simulink model "platformController"  (R2025b)
settings: Solver=FixedStepDiscrete  StartTime=0.0  StopTime=10  FixedStep=1/1000  RelTol=1e-3
InitFcn:
  | plant_parameters;
  | fluid_constants;
undefined symbols (not defined in the file or in its folder): DiscIntNeverNeededParam, mass, mission_mode, platform_targets
libraries: simulink x12, slpidlib x3, eeGeneralControl x1
settings Model: Creator=karadeli  LastModifiedBy=karadeli
settings OptimizationCC: DefaultParameterBehavior=Inlined  UseDivisionForNetSlopeComputation=on  GainParamInheritBuiltInType=on  UseFloatMulNetSlope=on  InlineInvariantSignals=on  PassReuseOutputArgsAs=Individual arguments  ZeroExternalMemoryAtStartup=off  ZeroInternalMemoryAtStartup=off  NoFixptDivByZeroProtection=on  EfficientFloat2IntCast=on  LifeSpan=1  OptimizeBlockOrder=speed  DifferentSizesBufferReuse=on  EfficientTunableParamExpr=on
settings DebuggingCC: ParameterTunabilityLossMsg=error
settings HardwareCC: ProdBitPerPointer=32.0  ProdBitPerSizeT=32.0  ProdBitPerPtrDiffT=32.0  ProdLargestAtomicInteger=Long  ProdLargestAtomicFloat=Double  ProdWordSize=32.0  ProdLongLongMode=on  ProdHWDeviceType=ARM Compatible->ARM Cortex-M
settings SFSimCC: MATLABDynamicMemAlloc=off
settings RTWCC: SystemTargetFile=ert.tlc  GenCodeOnly=on  TemplateMakefile=ert_default_tmf  TargetLang=C++  Description=Embedded Coder
settings CodeAppCC: ForceParamTrailComments=on  IgnoreCustomStorageClasses=off  OperatorAnnotations=on  SimulinkDataObjDesc=on  SFDataObjDesc=on  CustomSymbolStrGlobalVar=rt$N$M  CustomSymbolStrType=$N$M  CustomSymbolStrFcn=$N$M$F  CustomSymbolStrMacro=$N$M  InsertBlockDesc=on
settings ERTTargetCC: RootIOFormat=Structure reference  ERTCustomFileTemplate=example_file_process.tlc  ERTFilePackagingFormat=CompactWithDataFile  TargetLangStandard=C++11 (ISO)  GenerateSampleERTMain=on  IncludeMdlTerminateFcn=off  CombineSignalStateStructs=on  SupportAbsoluteTime=off  CodeInterfacePackaging=C++ class  SubcomponentCodeInterfacePackaging=C++ class  SupportNonFinite=off  SupportComplex=off  SupportNonInlinedSFcns=on

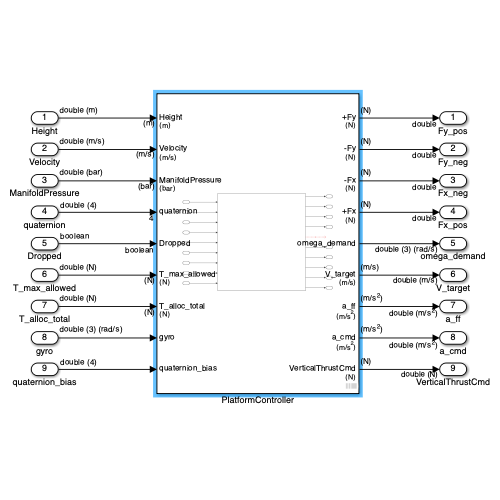
[thumbnail: Simulink's stored preview of the top-level diagram]
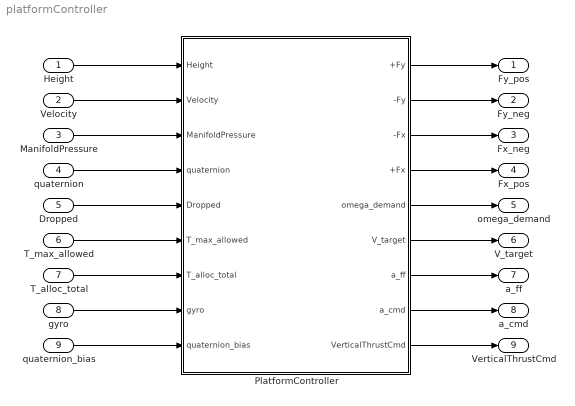
== system platformController ==
  Height : Inport  Unit=m
  Velocity : Inport  Port=2  Unit=m/s
  ManifoldPressure : Inport  Port=3  Unit=bar
  quaternion : Inport  Port=4  PortDimensions=4
  Dropped : Inport  Port=5  OutDataTypeStr=boolean
  T_max_allowed : Inport  Port=6  Unit=N
  T_alloc_total : Inport  Port=7  Unit=N
  gyro : Inport  Port=8
  quaternion_bias : Inport  Port=9  PortDimensions=4
  PlatformController : Subsystem
  Fy_pos : Outport
  Fy_neg : Outport  Port=2
  Fx_neg : Outport  Port=3
  Fx_pos : Outport  Port=4
  omega_demand : Outport  Port=5
  V_target : Outport  Port=6  Unit=m/s
  a_ff : Outport  Port=7  Unit=m/s^2
  a_cmd : Outport  Port=8  Unit=m/s^2
  VerticalThrustCmd : Outport  Port=9  Unit=N
  wires:
  T_max_allowed/1 -> PlatformController/6(T_max_allowed)
  T_alloc_total/1 -> PlatformController/7(T_alloc_total)
  Height/1 -> PlatformController/1(Height)
  Velocity/1 -> PlatformController/2(Velocity)
  quaternion/1 -> PlatformController/4(quaternion)
  ManifoldPressure/1 -> PlatformController/3(ManifoldPressure)
  Dropped/1 -> PlatformController/5(Dropped)
  gyro/1 -> PlatformController/8(gyro)
  PlatformController/5(omega_demand) -> omega_demand/1
  PlatformController/4(+Fx) -> Fx_pos/1
  PlatformController/3(-Fx) -> Fx_neg/1
  PlatformController/2(-Fy) -> Fy_neg/1
  PlatformController/1(+Fy) -> Fy_pos/1
  quaternion_bias/1 -> PlatformController/9(quaternion_bias)
  PlatformController/6(V_target) -> V_target/1
  PlatformController/9(VerticalThrustCmd) -> VerticalThrustCmd/1
  PlatformController/8(a_cmd) -> a_cmd/1
  PlatformController/7(a_ff) -> a_ff/1

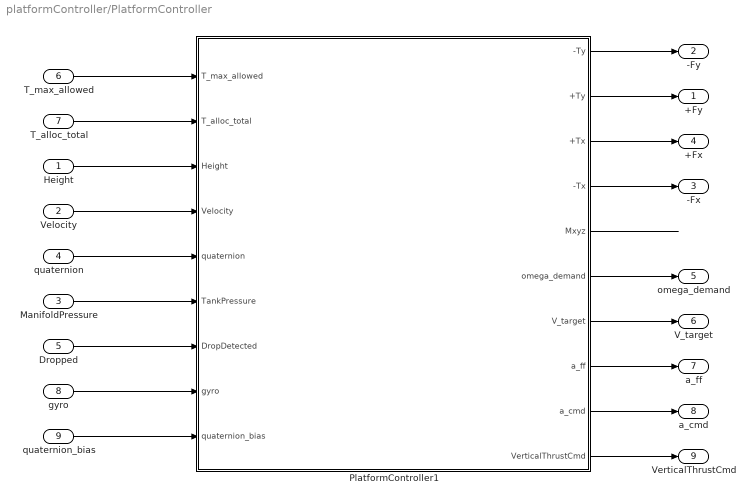
== system platformController/PlatformController ==
  Height : Inport  Unit=m
  Velocity : Inport  Port=2  Unit=m/s
  ManifoldPressure : Inport  Port=3  Unit=bar
  quaternion : Inport  Port=4  PortDimensions=4
  Dropped : Inport  Port=5  OutDataTypeStr=boolean
  T_max_allowed : Inport  Port=6  Unit=N
  T_alloc_total : Inport  Port=7  Unit=N
  gyro : Inport  Port=8
  quaternion_bias : Inport  Port=9
  PlatformController1 : Subsystem
  +Fy : Outport  Unit=N
  -Fy : Outport  Port=2  Unit=N
  -Fx : Outport  Port=3  Unit=N
  +Fx : Outport  Port=4  Unit=N
  omega_demand : Outport  Port=5
  V_target : Outport  Port=6  Unit=m/s
  a_ff : Outport  Port=7  Unit=m/s^2
  a_cmd : Outport  Port=8  Unit=m/s^2
  VerticalThrustCmd : Outport  Port=9  Unit=N
  wires:
  PlatformController1/1(-Ty) -> -Fy/1
  Height/1 -> PlatformController1/3(Height)
  gyro/1 -> PlatformController1/8(gyro)
  PlatformController1/6(omega_demand) -> omega_demand/1
  PlatformController1/5(Mxyz) -> ?
  Dropped/1 -> PlatformController1/7(DropDetected)
  T_alloc_total/1 -> PlatformController1/2(T_alloc_total)
  PlatformController1/2(+Ty) -> +Fy/1
  PlatformController1/4(-Tx) -> -Fx/1
  T_max_allowed/1 -> PlatformController1/1(T_max_allowed)
  quaternion/1 -> PlatformController1/5(quaternion)
  Velocity/1 -> PlatformController1/4(Velocity)
  ManifoldPressure/1 -> PlatformController1/6(TankPressure)
  PlatformController1/3(+Tx) -> +Fx/1
  quaternion_bias/1 -> PlatformController1/9(quaternion_bias)
  PlatformController1/7(V_target) -> V_target/1
  PlatformController1/8(a_ff) -> a_ff/1
  PlatformController1/9(a_cmd) -> a_cmd/1
  PlatformController1/10(VerticalThrustCmd) -> VerticalThrustCmd/1

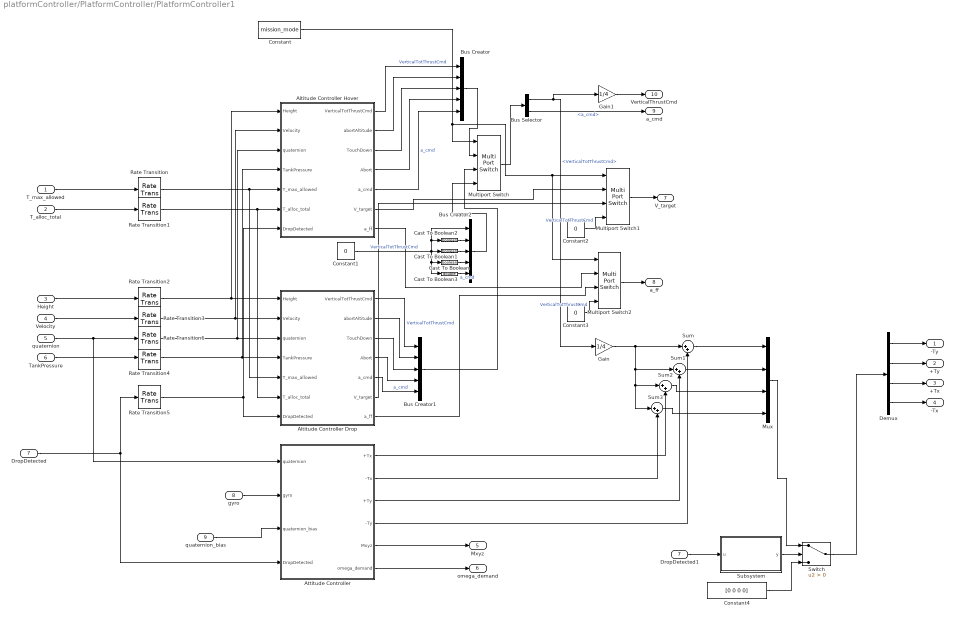
== system platformController/PlatformController/PlatformController1 ==
  T_max_allowed : Inport
  T_alloc_total : Inport  Port=2
  Height : Inport  Port=3
  Velocity : Inport  Port=4
  quaternion : Inport  Port=5
  TankPressure : Inport  Port=6
  DropDetected : Inport  Port=7
  gyro : Inport  Port=8  Unit=rad/s  PortDimensions=3
  quaternion_bias : Inport  Port=9
  Altitude Controller Drop : Subsystem
  Altitude Controller Hover : Subsystem
  Attitude Controller : Subsystem
  Bus Creator : BusCreator  Inputs=5
  Bus Creator1 : BusCreator  Inputs=5
  Bus Creator2 : BusCreator  Inputs=5
  Bus Selector : BusSelector  OutputSignals=VerticalTotThrustCmd,a_cmd
  Cast To Boolean : DataTypeConversion  OutDataTypeStr=boolean  SaturateOnIntegerOverflow=off  RndMeth=Floor
  Cast To Boolean1 : DataTypeConversion  OutDataTypeStr=boolean  SaturateOnIntegerOverflow=off  RndMeth=Floor
  Cast To Boolean2 : DataTypeConversion  OutDataTypeStr=boolean  SaturateOnIntegerOverflow=off  RndMeth=Floor
  Cast To Boolean3 : DataTypeConversion  OutDataTypeStr=double  SaturateOnIntegerOverflow=off  RndMeth=Floor
  Constant : Constant  Value=mission_mode  OutDataTypeStr=Enum: mission_modes
  Constant1 : Constant  Value=0
  Constant2 : Constant  Value=0
  Constant3 : Constant  Value=0
  Constant4 : Constant  Value=[0 0 0 0]
  Demux : Demux
  DropDetected1 : InportShadow  Port=7
  Gain : Gain  Gain=1/4
  Gain1 : Gain  Gain=1/4
  Multiport Switch : MultiPortSwitch  DataPortOrder=Specify indices  DataPortIndices={mission_modes.HOVER, mission_modes.DROP}  DataPortForDefault=Additional data port  SaturateOnIntegerOverflow=off  InputSameDT=off
  Multiport Switch1 : MultiPortSwitch  DataPortOrder=Specify indices  DataPortIndices={mission_modes.HOVER, mission_modes.DROP}  DataPortForDefault=Additional data port  SaturateOnIntegerOverflow=off  InputSameDT=off
  Multiport Switch2 : MultiPortSwitch  DataPortOrder=Specify indices  DataPortIndices={mission_modes.HOVER, mission_modes.DROP}  DataPortForDefault=Additional data port  SaturateOnIntegerOverflow=off  InputSameDT=off
  Mux : Mux
  Rate Transition{,1..6} (7 alike) : RateTransition  OutPortSampleTime=1/50
  Subsystem : Subsystem  mask{t_close=5}
  Sum{,1..3} (4 alike) : Sum  Inputs=|++
  Switch : Switch  Criteria=u2 > Threshold  SaturateOnIntegerOverflow=off  InputSameDT=off
  -Ty : Outport
  +Ty : Outport  Port=2
  +Tx : Outport  Port=3
  -Tx : Outport  Port=4
  Mxyz : Outport  Port=5
  omega_demand : Outport  Port=6
  V_target : Outport  Port=7
  a_ff : Outport  Port=8
  a_cmd : Outport  Port=9
  VerticalThrustCmd : Outport  Port=10
  wires:
  Cast To Boolean1/1 -> Bus Creator2/3
  T_alloc_total/1 -> Rate Transition1/1
  Sum2/1 -> Mux/3
  T_max_allowed/1 -> Rate Transition/1
  Altitude Controller Hover/2(abortAltitude) -> Bus Creator/2
  Multiport Switch/1 -> Bus Selector/1
  Cast To Boolean/1 -> Bus Creator2/4
  Altitude Controller Hover/3(TouchDown) -> Bus Creator/3
  Attitude Controller/2(-Tx) -> Sum3/2
  quaternion/1 -> Rate Transition6/1, Attitude Controller/1(quaternion)
  Height/1 -> Rate Transition2/1
  Velocity/1 -> Rate Transition3/1
  Cast To Boolean3/1 -> Bus Creator2/5  "a_cmd"
  gyro/1 -> Attitude Controller/2(gyro)
  Altitude Controller Hover/1(VerticalTotThrustCmd) -> Bus Creator/1  "VerticalTotThrustCmd"
  Gain/1 -> Sum/1, Sum1/1, Sum3/1, Sum2/1
  Bus Selector/1 -> Gain1/1, Gain/1  "<VerticalTotThrustCmd>"
  TankPressure/1 -> Rate Transition4/1
  Altitude Controller Drop/4(Abort) -> Bus Creator1/4
  Constant1/1 -> Cast To Boolean1/1, Cast To Boolean/1, Cast To Boolean3/1, Cast To Boolean2/1, Bus Creator2/1  "VerticalTotThrustCmd"
  Attitude Controller/1(+Tx) -> Sum2/2
  Attitude Controller/3(+Ty) -> Sum1/2
  Altitude Controller Drop/1(VerticalTotThrustCmd) -> Bus Creator1/1  "VerticalTotThrustCmd"
  Bus Creator/1 -> Multiport Switch/2
  Attitude Controller/4(-Ty) -> Sum/2
  Bus Creator1/1 -> Multiport Switch/3
  Altitude Controller Hover/4(Abort) -> Bus Creator/4
  DropDetected/1 -> Rate Transition5/1, Attitude Controller/4(DropDetected)
  Altitude Controller Drop/3(TouchDown) -> Bus Creator1/3
  Sum/1 -> Mux/1
  Altitude Controller Drop/2(abortAltitude) -> Bus Creator1/2
  Altitude Controller Hover/5(a_cmd) -> Bus Creator/5  "a_cmd"
  Cast To Boolean2/1 -> Bus Creator2/2
  Constant/1 -> Multiport Switch/1, Multiport Switch1/1, Multiport Switch2/1
  Bus Creator2/1 -> Multiport Switch/4
  Altitude Controller Drop/5(a_cmd) -> Bus Creator1/5  "a_cmd"
  Sum1/1 -> Mux/2
  Sum3/1 -> Mux/4
  Attitude Controller/5(Mxyz) -> Mxyz/1
  Rate Transition/1 -> Altitude Controller Drop/5(T_max_allowed), Altitude Controller Hover/5(T_max_allowed)
  Rate Transition1/1 -> Altitude Controller Drop/6(T_alloc_total), Altitude Controller Hover/6(T_alloc_total)
  Rate Transition2/1 -> Altitude Controller Hover/1(Height), Altitude Controller Drop/1(Height)
  Rate Transition3/1 -> Altitude Controller Hover/2(Velocity), Altitude Controller Drop/2(Velocity)
  Rate Transition4/1 -> Altitude Controller Hover/4(TankPressure), Altitude Controller Drop/4(TankPressure)
  Rate Transition5/1 -> Altitude Controller Hover/7(DropDetected), Altitude Controller Drop/7(DropDetected)
  Rate Transition6/1 -> Altitude Controller Drop/3(quaternion), Altitude Controller Hover/3(quaternion)
  Attitude Controller/6(omega_demand) -> omega_demand/1
  quaternion_bias/1 -> Attitude Controller/3(quaternion_bias)
  Altitude Controller Hover/6(V_target) -> Multiport Switch1/2
  Altitude Controller Drop/6(V_target) -> Multiport Switch1/3
  Constant2/1 -> Multiport Switch1/4  "VerticalTotThrustCmd"
  Multiport Switch1/1 -> V_target/1
  Constant3/1 -> Multiport Switch2/4  "VerticalTotThrustCmd"
  Multiport Switch2/1 -> a_ff/1
  Altitude Controller Hover/7(a_ff) -> Multiport Switch2/2
  Altitude Controller Drop/7(a_ff) -> Multiport Switch2/3
  Bus Selector/2 -> a_cmd/1  "<a_cmd>"
  Gain1/1 -> VerticalThrustCmd/1
  DropDetected1/1 -> Subsystem/1(u)
  Subsystem/1(y) -> Switch/2
  Constant4/1 -> Switch/3
  Demux/2 -> +Ty/1
  Demux/4 -> -Tx/1
  Demux/3 -> +Tx/1
  Demux/1 -> -Ty/1
  Mux/1 -> Switch/1
  Switch/1 -> Demux/1

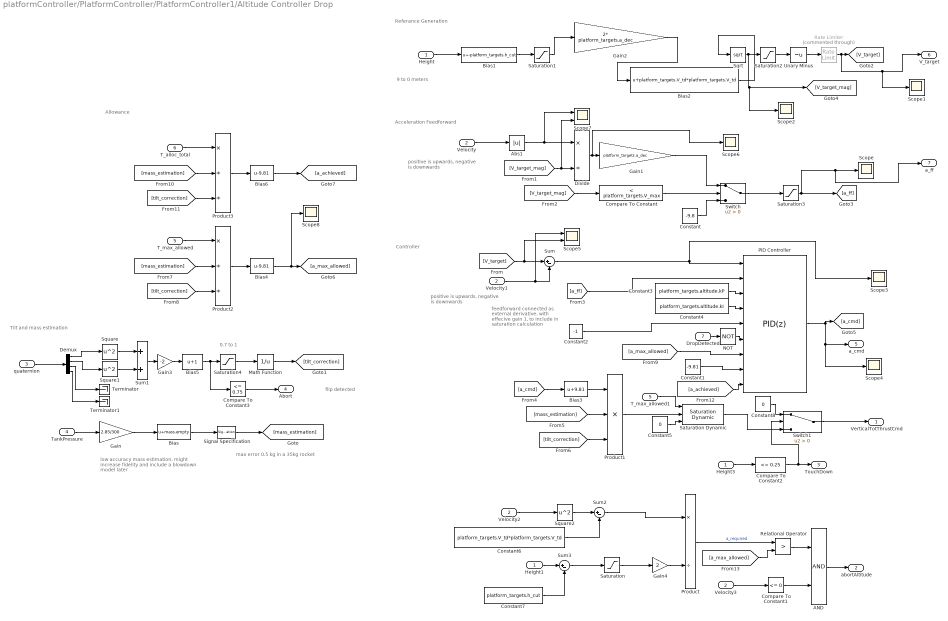
== system platformController/PlatformController/PlatformController1/Altitude Controller Drop ==
  note: flip detected
  note: max error 0.5 kg in a 35kg rocket
  note: 0.7 to 1
  note: Allowance
  note: Controller
  note: feedforward connected as external derivative, with effecive gain 1, to include in saturation calculation
  note: Tilt and mass estimation
  note: Acceleration Feedforward
  note: Referance Generation
  note: 9 to 0 meters
  note: low accuracy mass estimation, might increase fidelity and include a blowdown model later
  note: positive is upwards, negative is downwards
  note: positive is upwards, negative is downwards
  Height : Inport
  Velocity : Inport  Port=2
  quaternion : Inport  Port=3
  TankPressure : Inport  Port=4  Unit=bar
  T_max_allowed : Inport  Port=5  Unit=N
  T_alloc_total : Inport  Port=6
  DropDetected : Inport  Port=7
  AND : Logic  AllPortsSameDT=off  OutDataTypeStr=boolean
  Abs1 : Abs  SaturateOnIntegerOverflow=off
  Bias : Bias  Bias=mass.empty  SaturateOnIntegerOverflow=off
  Bias1 : Bias  Bias=-platform_targets.h_cut  SaturateOnIntegerOverflow=off
  Bias2 : Bias  Bias=platform_targets.V_td*platform_targets.V_td  SaturateOnIntegerOverflow=off
  Bias3 : Bias  Bias=9.81  SaturateOnIntegerOverflow=off
  Bias4 : Bias  Bias=-9.81  SaturateOnIntegerOverflow=off
  Bias5 : Bias  Bias=1  SaturateOnIntegerOverflow=off
  Bias6 : Bias  Bias=-9.81  SaturateOnIntegerOverflow=off
  Compare To Constant : simulink/Logic and Bit Operations/Compare To Constant  relop=<  const=platform_targets.V_max  OutDataTypeStr=boolean
  Compare To Constant1 : simulink/Logic and Bit Operations/Compare To Constant  relop=<=  const=0  OutDataTypeStr=boolean
  Compare To Constant2 : simulink/Logic and Bit Operations/Compare To Constant  relop=<=  const=0.25  OutDataTypeStr=boolean
  Compare To Constant3 : simulink/Logic and Bit Operations/Compare To Constant  relop=<=  const=0.75  OutDataTypeStr=boolean
  Constant : Constant  Value=-9.8
  Constant1 : Constant  Value=-9.81
  Constant2 : Constant  Value=-1
  Constant3 : Constant  Value=platform_targets.altitude.kP
  Constant4 : Constant  Value=platform_targets.altitude.kI
  Constant5 : Constant  Value=0
  Constant6 : Constant  Value=platform_targets.V_td*platform_targets.V_td
  Constant7 : Constant  Value=platform_targets.h_cut
  Constant8 : Constant  Value=0
  Demux : Demux
  Divide : Product  Inputs=*/
  Gain : Gain  Gain=2.85/300
  Gain1 : Gain  Gain=platform_targets.a_dec
  Gain2 : Gain  Gain=2* platform_targets.a_dec
  Gain3 : Gain  Gain=-2
  Gain4 : Gain  Gain=2
  Height1 : InportShadow
  Height3 : InportShadow
  Math Function : Math  Operator=reciprocal
  NOT : Logic  Operator=NOT  IconShape=distinctive  AllPortsSameDT=off  OutDataTypeStr=boolean
  PID Controller : slpidlib/PID Controller  Controller=PID  Form=Parallel  TimeDomain=Discrete-time  UseExternalTs=off  SampleTime=-1  IntegratorMethod=Forward Euler  FilterMethod=Forward Euler  ControllerParametersSource=external  P=1  I=1  UseKiTs=off  D=platform_targets.Ts  UseExternalDerivativeSource=on  N=100  UseFilter=off  TunerSelectOption=Frequency Response Based  InitialConditionSource=internal  InitialConditionForIntegrator=0  InitialConditionForFilter=0  DifferentiatorICPrevScaledInput=0  ExternalReset=level  TrackingMode=on  Kt=1  LimitOutput=on  SatLimitsSource=external  UpperSaturationLimit=inf  LowerSaturationLimit=-inf  LinearizeAsGain=on  AntiWindupMode=clamping  Kb=1  LimitIntegrator=on  UpperIntegratorSaturationLimit=3  LowerIntegratorSaturationLimit=-3  POutMin=[]  POutMax=[]  IOutMin=[]  IOutMax=[]  DOutMin=[]  DOutMax=[]  NOutMin=[]  NOutMax=[]  SumOutMin=[]  SumOutMax=[]  SaturationOutMin=[]  SaturationOutMax=[]  PParamMin=[]  PParamMax=[]  IParamMin=[]  IParamMax=[]  DParamMin=[]  DParamMax=[]  NParamMin=[]  NParamMax=[]  KbParamMin=[]  KbParamMax=[]  KtParamMin=[]  KtParamMax=[]  KbOutMin=[]  KbOutMax=[]  KtOutMin=[]  KtOutMax=[]  IntegratorOutMin=[]  IntegratorOutMax=[]  FilterOutMin=[]  FilterOutMax=[]  SumI1OutMin=[]  SumI1OutMax=[]  SumI2OutMin=[]  SumI2OutMax=[]  SumI3OutMin=[]  SumI3OutMax=[]  SumI4OutMin=[]  SumI4OutMax=[]  SumDOutMin=[]  SumDOutMax=[]  DifferentiatorOutMin=[]  DifferentiatorOutMax=[]  FilterDiffOutCoefMin=[]  FilterDiffOutCoefMax=[]  ReciprocalOutMin=[]  ReciprocalOutMax=[]  SumDenOutMin=[]  SumDenOutMax=[]  SumNumOutMin=[]  SumNumOutMax=[]  DivideOutMin=[]  DivideOutMax=[]  UdiffTsProdOutMin=[]  UdiffTsProdOutMax=[]  NTsProdOutMin=[]  NTsProdOutMax=[]  UintegralTsProdOutMin=[]  UintegralTsProdOutMax=[]  UngainTsProdOutMin=[]  UngainTsProdOutMax=[]  ClampingZeroOutDataTypeStr=Inherit: Inherit via back propagation  ClampingZeroOutMin=[]  ClampingZeroOutMax=[]  FilterDenConstantOutDataTypeStr=Inherit: Inherit via back propagation  FilterDenConstantOutMin=[]  FilterDenConstantOutMax=[]  PCopyOutDataTypeStr=Inherit: Inherit via back propagation  PCopyOutMin=[]  PCopyOutMax=[]  NCopyOutDataTypeStr=Inherit: Inherit via back propagation  NCopyOutMin=[]  NCopyOutMax=[]  IntegratorContinuousStateAttributes=''  IntegratorStateMustResolveToSignalObject=off  IntegratorRTWStateStorageClass=Auto  FilterContinuousStateAttributes=''  FilterStateMustResolveToSignalObject=off  FilterRTWStateStorageClass=Auto  ParallelPVariant=ExternalParameters  IdealPVariant=Disabled  IVariant=ExternalParameters  DVariant=ExternalParameters  IntegratorVariant=Discrete  SatVariant=External  AWVariant=DiscClampingParallel  PCopyVariant=Disabled  TRVariant=Enabled  FdbkBlocksVariant=Forward  IdealPFdbkVariant=Disabled  SatFdbkVariant=Disabled  DerivativeFilterVariant=Passthrough  NVariant=Passthrough  NCopyVariant=Disabled_SignalSpec  FilterICVariant=Disabled  IntegratorICVariant=InternalICs  ExternalResetVariant=ExternalReset  TRSumVariant=TrackingMode  SumFdbkVariant=Disabled  SumVariant=Sum_PID  TsampFilterVariant=InternalTs  TsampNgainVariant=Passthrough  TsampIntegralVariant=Disabled_SignalSpec  ExternalSaturationOutDataTypeStr=Inherit: Same as second input  DerivativeSourceVariant=ExternalYdot  PreIntVariant=InternalPreInt
  Product : Product  Inputs=*/
  Product1 : Product  Inputs=3
  Product2 : Product  Inputs=*//
  Product3 : Product  Inputs=*//
  Rate Limiter : RateLimiter  Commented=through  RisingSlewLimit=1.5*platform_targets.a_dec  FallingSlewLimit=-1.5*platform_targets.a_dec  SampleTimeMode=inherited
  Relational Operator : RelationalOperator  Operator=>  OutDataTypeStr=boolean  RndMeth=Simplest  InputSameDT=off
  Saturation : Saturate  UpperLimit=0.1  LowerLimit=-inf
  Saturation Dynamic : simulink/Discontinuities/Saturation Dynamic  OutMin=[]  OutMax=[]  OutDataTypeStr=Inherit: Same as second input  OutDataType=fixdt(1, 16)  OutScaling=2^-10  DoSatur=off
  Saturation1 : Saturate  UpperLimit=inf  LowerLimit=0
  Saturation2 : Saturate  UpperLimit=platform_targets.V_max  LowerLimit=-inf
  Saturation3 : Saturate  UpperLimit=platform_targets.a_dec  LowerLimit=-inf
  Saturation4 : Saturate  UpperLimit=1  LowerLimit=0.7
  Scope{,1..4,6,8} (7 alike) : Scope
      Scope settings: ActiveDisplayYMinimum=-11.775  ActiveDisplayYMaximum=7.975
      Scope1 settings: ActiveDisplayYMinimum=-1  ActiveDisplayYMaximum=1  DataLoggingVariableName=ScopeData2
      Scope2 settings: ActiveDisplayYMinimum=-1.827770577815089  ActiveDisplayYMaximum=17.449935200335805  DataLoggingVariableName=ScopeData3
      Scope3 settings: ActiveDisplayYMinimum=-1  ActiveDisplayYMaximum=1  DataLoggingVariableName=ScopeData5
      Scope4 settings: ActiveDisplayYMinimum=-11.845500622839467  ActiveDisplayYMaximum=8.5095056055552  DataLoggingVariableName=ScopeData6
      Scope6 settings: ActiveDisplayYMinimum=-2.8207729738075158  ActiveDisplayYMaximum=25.386956764267644  DataLoggingVariableName=ScopeData10
      Scope8 settings: ActiveDisplayYMinimum=1.4571466713688759  ActiveDisplayYMaximum=13.020751190028783  DataLoggingVariableName=ScopeData17
  Scope5 : Scope  NumInputPorts=2
      settings: ActiveDisplayYMinimum=-11.352374051095602  ActiveDisplayYMaximum=1.2613748945661778  DataLoggingVariableName=ScopeData9
  Scope7 : Scope  NumInputPorts=2
      settings: ActiveDisplayYMinimum=-1  ActiveDisplayYMaximum=1  DataLoggingVariableName=ScopeData11
  Signal Specification : SignalSpecification  Unit=kg
  Sqrt : Sqrt
  Square : Math  Operator=square
  Square1 : Math  Operator=square
  Square2 : Math  Operator=square
  Sum : Sum  Inputs=|+-
  Sum1 : Sum  Inputs=2
  Sum2 : Sum  Inputs=|+-
  Sum3 : Sum  Inputs=|+-
  Switch : Switch  Criteria=u2 > Threshold  SaturateOnIntegerOverflow=off  InputSameDT=off
  Switch1 : Switch  Criteria=u2 > Threshold  SaturateOnIntegerOverflow=off  InputSameDT=off
  T_max_allowed1 : InportShadow  Port=5  Unit=N
  Terminator : Terminator
  Terminator1 : Terminator
  Unary Minus : UnaryMinus
  Velocity1 : InportShadow  Port=2
  Velocity2 : InportShadow  Port=2
  Velocity3 : InportShadow  Port=2
  VerticalTotThrustCmd : Outport  Unit=N
  abortAltitude : Outport  Port=2
  TouchDown : Outport  Port=3
  Abort : Outport  Port=4
  a_cmd : Outport  Port=5  Unit=m/s^2
  V_target : Outport  Port=6
  a_ff : Outport  Port=7
  wires:
  Constant4/1 -> PID Controller/4
  Constant3/1 -> PID Controller/3
  [a_achieved] -> PID Controller/9
  Saturation3/1 -> [a_ff], a_ff/1, Scope/1
  Compare To Constant3/1 -> Abort/1
  TankPressure/1 -> Gain/1
  Gain/1 -> Bias/1
  Bias/1 -> Signal Specification/1
  Signal Specification/1 -> [mass_estimation]
  Math Function/1 -> [tilt_correction]
  Height/1 -> Bias1/1
  Bias1/1 -> Saturation1/1
  Saturation1/1 -> Gain2/1
  Gain2/1 -> Bias2/1
  Bias2/1 -> Sqrt/1
  Unary Minus/1 -> Rate Limiter/1
  Saturation2/1 -> Unary Minus/1
  [V_target_mag] -> Compare To Constant/1
  Compare To Constant/1 -> Switch/2
  Constant/1 -> Switch/3
  Switch/1 -> Saturation3/1
  Velocity/1 -> Abs1/1
  Sqrt/1 -> [V_target_mag], Scope2/1, Saturation2/1
  [V_target_mag] -> Divide/2, Scope7/2
  Abs1/1 -> Divide/1, Scope7/1
  Divide/1 -> Gain1/1, Scope6/1
  Gain1/1 -> Switch/1
  [V_target] -> Sum/1, Scope5/2
  Velocity1/1 -> Sum/2, Scope5/1
  Constant1/1 -> PID Controller/8
  [a_max_allowed] -> PID Controller/7
  Sum/1 -> PID Controller/1, Scope3/1
  [a_ff] -> PID Controller/2
  Constant2/1 -> PID Controller/5
  PID Controller/1 -> a_cmd/1, Scope4/1, [a_cmd]
  [a_cmd] -> Bias3/1
  Bias3/1 -> Product1/1
  [mass_estimation] -> Product1/2
  [tilt_correction] -> Product1/3
  Product1/1 -> Saturation Dynamic/2
  Switch1/1 -> VerticalTotThrustCmd/1
  Constant5/1 -> Saturation Dynamic/3
  [tilt_correction] -> Product2/3
  [mass_estimation] -> Product2/2
  T_max_allowed/1 -> Product2/1
  Product2/1 -> Bias4/1
  Bias4/1 -> [a_max_allowed], Scope8/1
  T_max_allowed1/1 -> Saturation Dynamic/1
  Saturation4/1 -> Math Function/1
  quaternion/1 -> Demux/1
  Demux/1 -> Square/1
  Demux/2 -> Square1/1
  Demux/3 -> Terminator/1
  Square/1 -> Sum1/1
  Square1/1 -> Sum1/2
  Sum1/1 -> Gain3/1
  Gain3/1 -> Bias5/1
  Bias5/1 -> Compare To Constant3/1, Saturation4/1
  T_alloc_total/1 -> Product3/1
  [mass_estimation] -> Product3/2
  Product3/1 -> Bias6/1
  [tilt_correction] -> Product3/3
  Bias6/1 -> [a_achieved]
  Rate Limiter/1 -> V_target/1, Scope1/1, [V_target]
  DropDetected/1 -> NOT/1
  NOT/1 -> PID Controller/6
  Velocity2/1 -> Square2/1
  Sum2/1 -> Product/1
  Square2/1 -> Sum2/1
  Constant6/1 -> Sum2/2
  Height1/1 -> Sum3/1
  Constant7/1 -> Sum3/2
  Sum3/1 -> Saturation/1
  Gain4/1 -> Product/2
  Saturation/1 -> Gain4/1
  Product/1 -> Relational Operator/1  "a_required"
  Relational Operator/1 -> AND/1
  [a_max_allowed] -> Relational Operator/2
  AND/1 -> abortAltitude/1
  Velocity3/1 -> Compare To Constant1/1
  Compare To Constant1/1 -> AND/2
  Demux/4 -> Terminator1/1
  Saturation Dynamic/1 -> Switch1/3
  Compare To Constant2/1 -> Switch1/2, TouchDown/1
  Height3/1 -> Compare To Constant2/1
  Constant8/1 -> Switch1/1

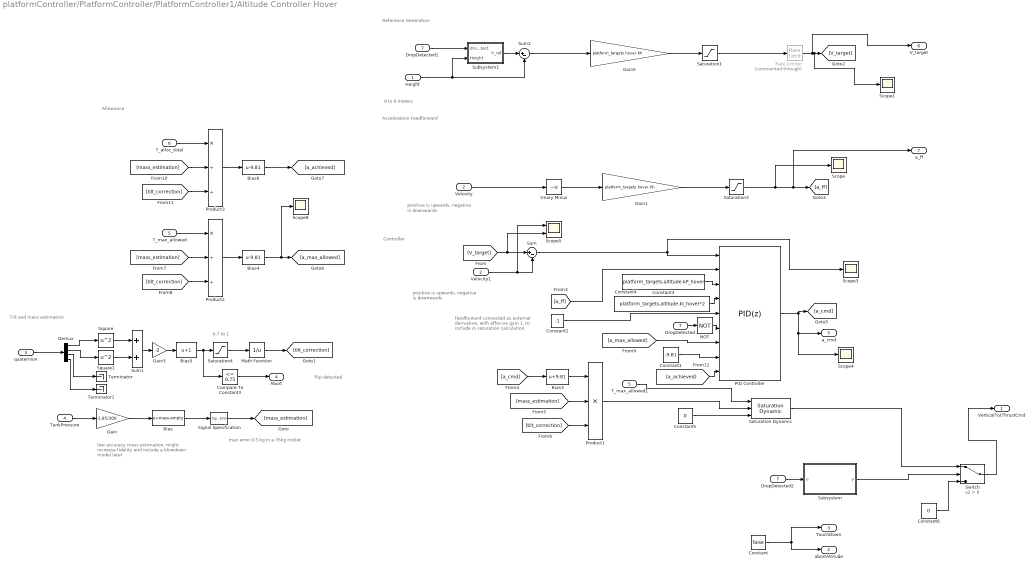
== system platformController/PlatformController/PlatformController1/Altitude Controller Hover ==
  note: positive is upwards, negative is downwards
  note: positive is upwards, negative is downwards
  note: low accuracy mass estimation, might increase fidelity and include a blowdown model later
  note: 9 to 0 meters
  note: Referance Generation
  note: Acceleration Feedforward
  note: Tilt and mass estimation
  note: feedforward connected as external derivative, with effecive gain 1, to include in saturation calculation
  note: Controller
  note: Allowance
  note: 0.7 to 1
  note: max error 0.5 kg in a 35kg rocket
  note: flip detected
  Height : Inport
  Velocity : Inport  Port=2
  quaternion : Inport  Port=3
  TankPressure : Inport  Port=4  Unit=bar
  T_max_allowed : Inport  Port=5  Unit=N
  T_alloc_total : Inport  Port=6
  DropDetected : Inport  Port=7
  Bias : Bias  Bias=mass.empty  SaturateOnIntegerOverflow=off
  Bias3 : Bias  Bias=9.81  SaturateOnIntegerOverflow=off
  Bias4 : Bias  Bias=-9.81  SaturateOnIntegerOverflow=off
  Bias5 : Bias  Bias=1  SaturateOnIntegerOverflow=off
  Bias6 : Bias  Bias=-9.81  SaturateOnIntegerOverflow=off
  Compare To Constant3 : simulink/Logic and Bit Operations/Compare To Constant  relop=<=  const=0.75  OutDataTypeStr=boolean
  Constant : Constant  Value=false
  Constant1 : Constant  Value=-9.81
  Constant2 : Constant  Value=-1
  Constant3 : Constant  Value=platform_targets.altitude.kP_hover
  Constant4 : Constant  Value=platform_targets.altitude.kI_hover*2
  Constant5 : Constant  Value=0
  Constant6 : Constant  Value=0
  Demux : Demux
  DropDetected1 : InportShadow  Port=7
  DropDetected2 : InportShadow  Port=7
  Gain : Gain  Gain=2.85/300
  Gain1 : Gain  Gain=platform_targets.hover.Kh
  Gain3 : Gain  Gain=-2
  Gain5 : Gain  Gain=platform_targets.hover.Kh
  Math Function : Math  Operator=reciprocal
  NOT : Logic  Operator=NOT  IconShape=distinctive  AllPortsSameDT=off  OutDataTypeStr=boolean
  PID Controller : slpidlib/PID Controller  Controller=PID  Form=Parallel  TimeDomain=Discrete-time  UseExternalTs=off  SampleTime=-1  IntegratorMethod=Forward Euler  FilterMethod=Forward Euler  ControllerParametersSource=external  P=1  I=1  UseKiTs=off  D=platform_targets.Ts  UseExternalDerivativeSource=on  N=100  UseFilter=off  TunerSelectOption=Frequency Response Based  InitialConditionSource=internal  InitialConditionForIntegrator=-9.81  InitialConditionForFilter=0  DifferentiatorICPrevScaledInput=0  ExternalReset=level  TrackingMode=on  Kt=1  LimitOutput=on  SatLimitsSource=external  UpperSaturationLimit=inf  LowerSaturationLimit=-inf  LinearizeAsGain=on  AntiWindupMode=clamping  Kb=1  LimitIntegrator=on  UpperIntegratorSaturationLimit=3  LowerIntegratorSaturationLimit=-10  POutMin=[]  POutMax=[]  IOutMin=[]  IOutMax=[]  DOutMin=[]  DOutMax=[]  NOutMin=[]  NOutMax=[]  SumOutMin=[]  SumOutMax=[]  SaturationOutMin=[]  SaturationOutMax=[]  PParamMin=[]  PParamMax=[]  IParamMin=[]  IParamMax=[]  DParamMin=[]  DParamMax=[]  NParamMin=[]  NParamMax=[]  KbParamMin=[]  KbParamMax=[]  KtParamMin=[]  KtParamMax=[]  KbOutMin=[]  KbOutMax=[]  KtOutMin=[]  KtOutMax=[]  IntegratorOutMin=[]  IntegratorOutMax=[]  FilterOutMin=[]  FilterOutMax=[]  SumI1OutMin=[]  SumI1OutMax=[]  SumI2OutMin=[]  SumI2OutMax=[]  SumI3OutMin=[]  SumI3OutMax=[]  SumI4OutMin=[]  SumI4OutMax=[]  SumDOutMin=[]  SumDOutMax=[]  DifferentiatorOutMin=[]  DifferentiatorOutMax=[]  FilterDiffOutCoefMin=[]  FilterDiffOutCoefMax=[]  ReciprocalOutMin=[]  ReciprocalOutMax=[]  SumDenOutMin=[]  SumDenOutMax=[]  SumNumOutMin=[]  SumNumOutMax=[]  DivideOutMin=[]  DivideOutMax=[]  UdiffTsProdOutMin=[]  UdiffTsProdOutMax=[]  NTsProdOutMin=[]  NTsProdOutMax=[]  UintegralTsProdOutMin=[]  UintegralTsProdOutMax=[]  UngainTsProdOutMin=[]  UngainTsProdOutMax=[]  ClampingZeroOutDataTypeStr=Inherit: Inherit via back propagation  ClampingZeroOutMin=[]  ClampingZeroOutMax=[]  FilterDenConstantOutDataTypeStr=Inherit: Inherit via back propagation  FilterDenConstantOutMin=[]  FilterDenConstantOutMax=[]  PCopyOutDataTypeStr=Inherit: Inherit via back propagation  PCopyOutMin=[]  PCopyOutMax=[]  NCopyOutDataTypeStr=Inherit: Inherit via back propagation  NCopyOutMin=[]  NCopyOutMax=[]  IntegratorContinuousStateAttributes=''  IntegratorStateMustResolveToSignalObject=off  IntegratorRTWStateStorageClass=Auto  FilterContinuousStateAttributes=''  FilterStateMustResolveToSignalObject=off  FilterRTWStateStorageClass=Auto  ParallelPVariant=ExternalParameters  IdealPVariant=Disabled  IVariant=ExternalParameters  DVariant=ExternalParameters  IntegratorVariant=Discrete  SatVariant=External  AWVariant=DiscClampingParallel  PCopyVariant=Disabled  TRVariant=Enabled  FdbkBlocksVariant=Forward  IdealPFdbkVariant=Disabled  SatFdbkVariant=Disabled  DerivativeFilterVariant=Passthrough  NVariant=Passthrough  NCopyVariant=Disabled_SignalSpec  FilterICVariant=Disabled  IntegratorICVariant=InternalICs  ExternalResetVariant=ExternalReset  TRSumVariant=TrackingMode  SumFdbkVariant=Disabled  SumVariant=Sum_PID  TsampFilterVariant=InternalTs  TsampNgainVariant=Passthrough  TsampIntegralVariant=Disabled_SignalSpec  ExternalSaturationOutDataTypeStr=Inherit: Same as second input  DerivativeSourceVariant=ExternalYdot  PreIntVariant=InternalPreInt
  Product1 : Product  Inputs=3
  Product2 : Product  Inputs=*//
  Product3 : Product  Inputs=*//
  Rate Limiter : RateLimiter  Commented=through  RisingSlewLimit=1.5*platform_targets.a_dec  FallingSlewLimit=-1.5*platform_targets.a_dec  SampleTimeMode=inherited
  Saturation Dynamic : simulink/Discontinuities/Saturation Dynamic  OutMin=[]  OutMax=[]  OutDataTypeStr=Inherit: Same as second input  OutDataType=fixdt(1, 16)  OutScaling=2^-10  DoSatur=off
  Saturation1 : Saturate  UpperLimit=platform_targets.hover.v_sat(2)  LowerLimit=platform_targets.hover.v_sat(1)
  Saturation3 : Saturate  UpperLimit=platform_targets.a_dec_low  LowerLimit=-9.81
  Saturation4 : Saturate  UpperLimit=1  LowerLimit=0.7
  Scope{,1,3..4,8} (5 alike) : Scope
      Scope settings: ActiveDisplayYMinimum=-4.8842151449601854  ActiveDisplayYMaximum=0.58928900764920311
      Scope1 settings: ActiveDisplayYMinimum=-1  ActiveDisplayYMaximum=1  DataLoggingVariableName=ScopeData2
      Scope3 settings: ActiveDisplayYMinimum=-1  ActiveDisplayYMaximum=1  DataLoggingVariableName=ScopeData5
      Scope4 settings: ActiveDisplayYMinimum=-11.845500622839467  ActiveDisplayYMaximum=8.5095056055552  DataLoggingVariableName=ScopeData6
      Scope8 settings: ActiveDisplayYMinimum=17.11972656665862  ActiveDisplayYMaximum=25.442656839268942  DataLoggingVariableName=ScopeData17
  Scope5 : Scope  NumInputPorts=2
      settings: ActiveDisplayYMinimum=-0.54393861343044725  ActiveDisplayYMaximum=2.5048820681589388  DataLoggingVariableName=ScopeData9
  Signal Specification : SignalSpecification  Unit=kg
  Square : Math  Operator=square
  Square1 : Math  Operator=square
  Subsystem : Subsystem  mask{t_close=5}
  Subsystem1 : Subsystem
  Sum : Sum  Inputs=|+-
  Sum1 : Sum  Inputs=2
  Sum2 : Sum  Inputs=|+-
  Switch : Switch  Criteria=u2 > Threshold  SaturateOnIntegerOverflow=off  InputSameDT=off
  T_max_allowed1 : InportShadow  Port=5  Unit=N
  Terminator : Terminator
  Terminator1 : Terminator
  Unary Minus : UnaryMinus
  Velocity1 : InportShadow  Port=2
  VerticalTotThrustCmd : Outport  Unit=N
  abortAltitude : Outport  Port=2
  TouchDown : Outport  Port=3
  Abort : Outport  Port=4
  a_cmd : Outport  Port=5  Unit=m/s^2
  V_target : Outport  Port=6
  a_ff : Outport  Port=7
  wires:
  Constant/1 -> abortAltitude/1, TouchDown/1
  Demux/4 -> Terminator1/1
  NOT/1 -> PID Controller/6
  DropDetected/1 -> NOT/1
  Bias6/1 -> [a_achieved]
  [tilt_correction] -> Product3/3
  Product3/1 -> Bias6/1
  [mass_estimation] -> Product3/2
  T_alloc_total/1 -> Product3/1
  Bias5/1 -> Saturation4/1, Compare To Constant3/1
  Gain3/1 -> Bias5/1
  Sum1/1 -> Gain3/1
  Square1/1 -> Sum1/2
  Square/1 -> Sum1/1
  Demux/3 -> Terminator/1
  Demux/2 -> Square1/1
  Demux/1 -> Square/1
  quaternion/1 -> Demux/1
  Saturation4/1 -> Math Function/1
  T_max_allowed1/1 -> Saturation Dynamic/1
  Bias4/1 -> Scope8/1, [a_max_allowed]
  Product2/1 -> Bias4/1
  T_max_allowed/1 -> Product2/1
  [mass_estimation] -> Product2/2
  [tilt_correction] -> Product2/3
  Constant5/1 -> Saturation Dynamic/3
  Saturation Dynamic/1 -> Switch/1
  Product1/1 -> Saturation Dynamic/2
  [tilt_correction] -> Product1/3
  [mass_estimation] -> Product1/2
  Bias3/1 -> Product1/1
  [a_cmd] -> Bias3/1
  PID Controller/1 -> [a_cmd], Scope4/1, a_cmd/1
  Constant2/1 -> PID Controller/5
  [a_ff] -> PID Controller/2
  Sum/1 -> Scope3/1, PID Controller/1
  [a_max_allowed] -> PID Controller/7
  Constant1/1 -> PID Controller/8
  Velocity1/1 -> Scope5/1, Sum/2
  [V_target] -> Scope5/2, Sum/1
  Velocity/1 -> Unary Minus/1
  Gain1/1 -> Saturation3/1
  Saturation1/1 -> Rate Limiter/1
  Gain5/1 -> Saturation1/1
  Math Function/1 -> [tilt_correction]
  Signal Specification/1 -> [mass_estimation]
  Bias/1 -> Signal Specification/1
  Gain/1 -> Bias/1
  TankPressure/1 -> Gain/1
  Compare To Constant3/1 -> Abort/1
  Saturation3/1 -> Scope/1, a_ff/1, [a_ff]
  [a_achieved] -> PID Controller/9
  Constant3/1 -> PID Controller/3
  Constant4/1 -> PID Controller/4
  Height/1 -> Subsystem1/2(Height), Sum2/2
  Sum2/1 -> Gain5/1
  Unary Minus/1 -> Gain1/1
  Rate Limiter/1 -> V_target/1, Scope1/1, [V_target]
  DropDetected1/1 -> Subsystem1/1(drop_detect)
  Subsystem1/1(h_ref) -> Sum2/1
  DropDetected2/1 -> Subsystem/1(u)
  Subsystem/1(y) -> Switch/2
  Constant6/1 -> Switch/3
  Switch/1 -> VerticalTotThrustCmd/1

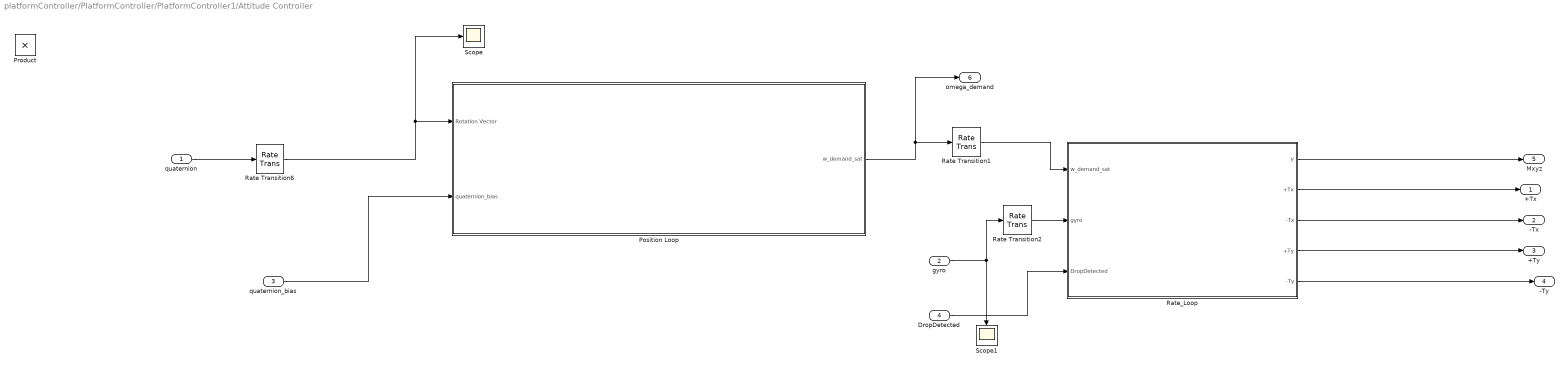
== system platformController/PlatformController/PlatformController1/Attitude Controller ==
  quaternion : Inport
  gyro : Inport  Port=2
  quaternion_bias : Inport  Port=3
  DropDetected : Inport  Port=4
  Position Loop : Subsystem
  Product : Product
  Rate Transition1 : RateTransition  OutPortSampleTime=1/200
  Rate Transition2 : RateTransition  OutPortSampleTime=1/200
  Rate Transition6 : RateTransition  OutPortSampleTime=1/100
  Rate_Loop : Subsystem
  Scope : Scope
      settings: ActiveDisplayYMinimum=-0.012499999999999997  ActiveDisplayYMaximum=0.1125  DataLoggingVariableName=ScopeData12
  Scope1 : Scope
      settings: ActiveDisplayYMinimum=-0.61375881480909644  ActiveDisplayYMaximum=1.2765015354334854  DataLoggingVariableName=ScopeData26
  +Tx : Outport
  -Tx : Outport  Port=2
  +Ty : Outport  Port=3
  -Ty : Outport  Port=4
  Mxyz : Outport  Port=5
  omega_demand : Outport  Port=6  Unit=rad/s  PortDimensions=3
  wires:
  quaternion/1 -> Rate Transition6/1
  Position Loop/1(w_demand_sat) -> omega_demand/1, Rate Transition1/1
  gyro/1 -> Scope1/1, Rate Transition2/1
  Rate_Loop/1(y) -> Mxyz/1
  Rate_Loop/2(+Tx) -> +Tx/1
  Rate_Loop/3(-Tx) -> -Tx/1
  Rate_Loop/4(+Ty) -> +Ty/1
  Rate_Loop/5(-Ty) -> -Ty/1
  Rate Transition1/1 -> Rate_Loop/1(w_demand_sat)
  Rate Transition2/1 -> Rate_Loop/2(gyro)
  Rate Transition6/1 -> Scope/1, Position Loop/1(Rotation Vector)
  DropDetected/1 -> Rate_Loop/3(DropDetected)
  quaternion_bias/1 -> Position Loop/2(quaternion_bias)

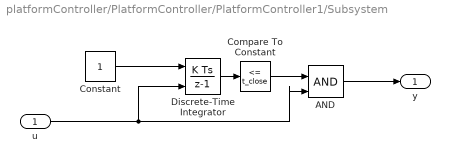
== system platformController/PlatformController/PlatformController1/Subsystem ==
  u : Inport
  AND : Logic  IconShape=distinctive  AllPortsSameDT=off  OutDataTypeStr=boolean
  Compare To Constant : simulink/Logic and Bit Operations/Compare To Constant  relop=<=  const=t_close  OutDataTypeStr=boolean
  Constant : Constant
  Discrete-Time Integrator : DiscreteIntegrator  ExternalReset=either  SampleTime=-1  ICPrevOutput=DiscIntNeverNeededParam  ICPrevScaledInput=DiscIntNeverNeededParam
  y : Outport
  wires:
  AND/1 -> y/1
  Constant/1 -> Discrete-Time Integrator/1
  u/1 -> Discrete-Time Integrator/2, AND/2
  Compare To Constant/1 -> AND/1
  Discrete-Time Integrator/1 -> Compare To Constant/1

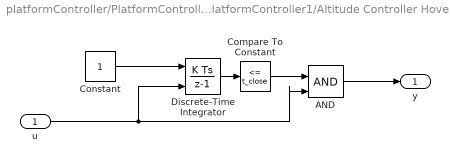
== system platformController/PlatformController/PlatformController1/Altitude Controller Hover/Subsystem ==
  u : Inport
  AND : Logic  IconShape=distinctive  AllPortsSameDT=off  OutDataTypeStr=boolean
  Compare To Constant : simulink/Logic and Bit Operations/Compare To Constant  relop=<=  const=t_close  OutDataTypeStr=boolean
  Constant : Constant
  Discrete-Time Integrator : DiscreteIntegrator  ExternalReset=either  SampleTime=-1  ICPrevOutput=DiscIntNeverNeededParam  ICPrevScaledInput=DiscIntNeverNeededParam
  y : Outport
  wires:
  AND/1 -> y/1
  Constant/1 -> Discrete-Time Integrator/1
  u/1 -> Discrete-Time Integrator/2, AND/2
  Compare To Constant/1 -> AND/1
  Discrete-Time Integrator/1 -> Compare To Constant/1

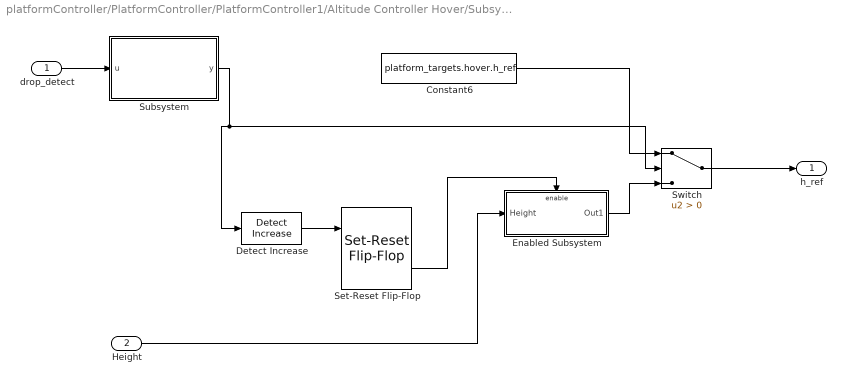
== system platformController/PlatformController/PlatformController1/Altitude Controller Hover/Subsystem1 ==
  drop_detect : Inport
  Height : Inport  Port=2
  Constant6 : Constant  Value=platform_targets.hover.h_ref
  Detect Increase : simulink/Logic and Bit Operations/Detect Increase  vinit=0.0  OutDataTypeStr=boolean
  Enabled Subsystem : Subsystem  TreatAsAtomicUnit=on
  Set-Reset Flip-Flop : eeGeneralControl/Set-Reset Flip-Flop  LabelModeActiveChoice=Discrete  UndefState=Set  Q0=0  Ts=-1
      settings: LibrarySourceBlock=ee_sl_lib/General Control/Set-Reset Flip-Flop
  Subsystem : Subsystem  mask{t_close=4}
  Switch : Switch  Criteria=u2 > Threshold  SaturateOnIntegerOverflow=off  InputSameDT=off
  h_ref : Outport
  wires:
  Enabled Subsystem/1(Out1) -> Switch/3
  Switch/1 -> h_ref/1
  Constant6/1 -> Switch/1
  Subsystem/1(y) -> Detect Increase/1, Switch/2
  Height/1 -> Enabled Subsystem/1(Height)
  Detect Increase/1 -> Set-Reset Flip-Flop/1
  Set-Reset Flip-Flop/2 -> Enabled Subsystem/Enable
  drop_detect/1 -> Subsystem/1(u)

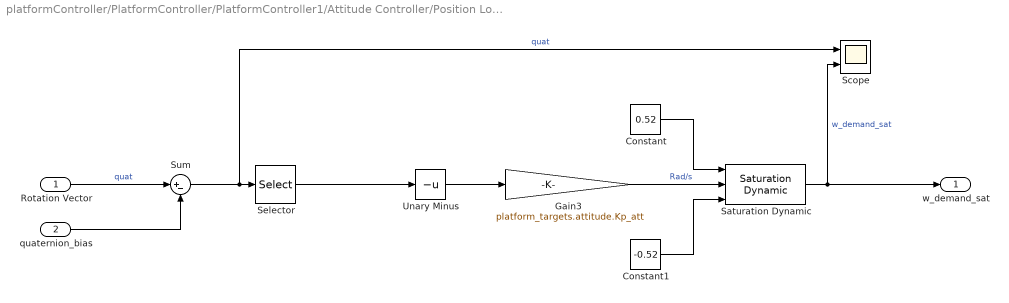
== system platformController/PlatformController/PlatformController1/Attitude Controller/Position Loop ==
  Rotation Vector : Inport
  quaternion_bias : Inport  Port=2
  Constant : Constant  Value=0.52
  Constant1 : Constant  Value=-0.52
  Gain3 : Gain  Gain=platform_targets.attitude.Kp_att
  Saturation Dynamic : simulink/Discontinuities/Saturation Dynamic  OutMin=[]  OutMax=[]  OutDataTypeStr=Inherit: Same as second input  OutDataType=fixdt(1, 16)  OutScaling=2^-10  DoSatur=off
  Scope : Scope  NumInputPorts=2
      settings: ActiveDisplayYMinimum=-0.69968634161992349  ActiveDisplayYMaximum=0.616400927563149  DataLoggingVariableName=ScopeData25
  Selector : Selector  InputPortWidth=4  IndexOptions=Index vector (dialog)  Indices=[1 2 3]  OutputSizes=1
  Sum : Sum  Inputs=|+-
  Unary Minus : UnaryMinus
  w_demand_sat : Outport
  wires:
  Constant1/1 -> Saturation Dynamic/3
  Constant/1 -> Saturation Dynamic/1
  Sum/1 -> Selector/1, Scope/1  "quat"
  Gain3/1 -> Saturation Dynamic/2  "Rad/s"
  Saturation Dynamic/1 -> w_demand_sat/1, Scope/2  "w_demand_sat"
  Selector/1 -> Unary Minus/1
  Unary Minus/1 -> Gain3/1
  Rotation Vector/1 -> Sum/1  "quat"
  quaternion_bias/1 -> Sum/2

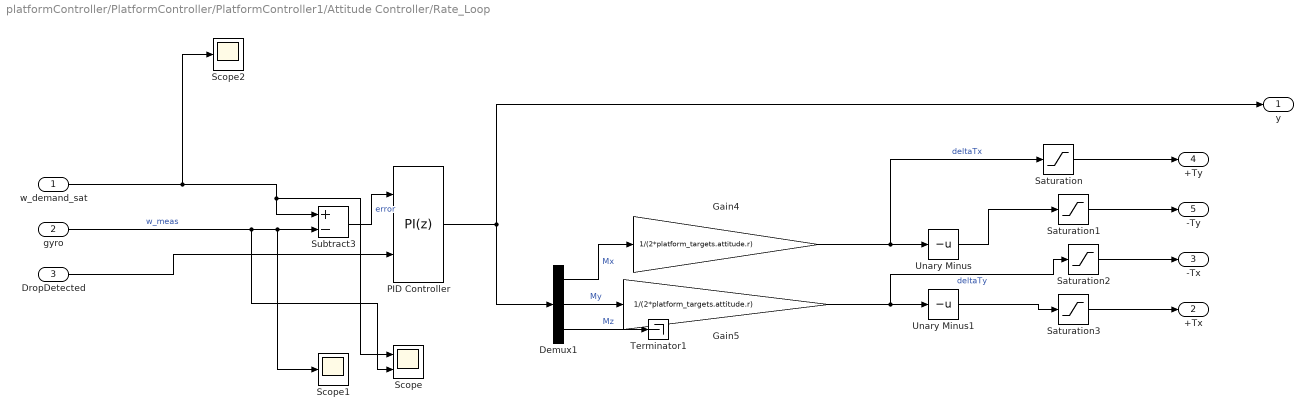
== system platformController/PlatformController/PlatformController1/Attitude Controller/Rate_Loop ==
  w_demand_sat : Inport
  gyro : Inport  Port=2
  DropDetected : Inport  Port=3
  Demux1 : Demux  Outputs=3
  Gain4 : Gain  Gain=1/(2*platform_targets.attitude.r)
  Gain5 : Gain  Gain=1/(2*platform_targets.attitude.r)
  PID Controller : slpidlib/PID Controller  Controller=PI  Form=Parallel  TimeDomain=Discrete-time  UseExternalTs=off  SampleTime=-1  IntegratorMethod=Forward Euler  FilterMethod=Forward Euler  ControllerParametersSource=internal  P=platform_targets.attitude.Kp_rate  I=platform_targets.attitude.Ki_rate  UseKiTs=off  D=0  UseExternalDerivativeSource=off  N=100  UseFilter=on  TunerSelectOption=Transfer Function Based (PID Tuner App)  InitialConditionSource=internal  InitialConditionForIntegrator=0  InitialConditionForFilter=0  DifferentiatorICPrevScaledInput=0  ExternalReset=rising  TrackingMode=off  Kt=1  LimitOutput=on  SatLimitsSource=internal  UpperSaturationLimit=16.5  LowerSaturationLimit=-16.5  LinearizeAsGain=on  AntiWindupMode=back-calculation  Kb=platform_targets.attitude.Ki_rate/platform_targets.attitude.Kp_rate  LimitIntegrator=on  UpperIntegratorSaturationLimit=16.5  LowerIntegratorSaturationLimit=-16.5  POutMin=[]  POutMax=[]  IOutMin=[]  IOutMax=[]  DOutMin=[]  DOutMax=[]  NOutMin=[]  NOutMax=[]  SumOutMin=[]  SumOutMax=[]  SaturationOutMin=[]  SaturationOutMax=[]  PParamMin=[]  PParamMax=[]  IParamMin=[]  IParamMax=[]  DParamMin=[]  DParamMax=[]  NParamMin=[]  NParamMax=[]  KbParamMin=[]  KbParamMax=[]  KtParamMin=[]  KtParamMax=[]  KbOutMin=[]  KbOutMax=[]  KtOutMin=[]  KtOutMax=[]  IntegratorOutMin=[]  IntegratorOutMax=[]  FilterOutMin=[]  FilterOutMax=[]  SumI1OutMin=[]  SumI1OutMax=[]  SumI2OutMin=[]  SumI2OutMax=[]  SumI3OutMin=[]  SumI3OutMax=[]  SumI4OutMin=[]  SumI4OutMax=[]  SumDOutMin=[]  SumDOutMax=[]  DifferentiatorOutMin=[]  DifferentiatorOutMax=[]  FilterDiffOutCoefMin=[]  FilterDiffOutCoefMax=[]  ReciprocalOutMin=[]  ReciprocalOutMax=[]  SumDenOutMin=[]  SumDenOutMax=[]  SumNumOutMin=[]  SumNumOutMax=[]  DivideOutMin=[]  DivideOutMax=[]  UdiffTsProdOutMin=[]  UdiffTsProdOutMax=[]  NTsProdOutMin=[]  NTsProdOutMax=[]  UintegralTsProdOutMin=[]  UintegralTsProdOutMax=[]  UngainTsProdOutMin=[]  UngainTsProdOutMax=[]  ClampingZeroOutDataTypeStr=Inherit: Inherit via back propagation  ClampingZeroOutMin=[]  ClampingZeroOutMax=[]  FilterDenConstantOutDataTypeStr=Inherit: Inherit via back propagation  FilterDenConstantOutMin=[]  FilterDenConstantOutMax=[]  PCopyOutDataTypeStr=Inherit: Inherit via back propagation  PCopyOutMin=[]  PCopyOutMax=[]  NCopyOutDataTypeStr=Inherit: Inherit via back propagation  NCopyOutMin=[]  NCopyOutMax=[]  IntegratorContinuousStateAttributes=''  IntegratorStateMustResolveToSignalObject=off  IntegratorRTWStateStorageClass=Auto  FilterContinuousStateAttributes=''  FilterStateMustResolveToSignalObject=off  FilterRTWStateStorageClass=Auto  ParallelPVariant=InternalParameters  IdealPVariant=Disabled  IVariant=InternalParameters  DVariant=Disabled  IntegratorVariant=Discrete  SatVariant=Enabled  AWVariant=BackCalculation  PCopyVariant=Disabled  TRVariant=Disabled  FdbkBlocksVariant=Forward  IdealPFdbkVariant=Disabled  SatFdbkVariant=Disabled  DerivativeFilterVariant=Disabled  NVariant=Disabled  NCopyVariant=Disabled_SignalSpec  FilterICVariant=Disabled  IntegratorICVariant=InternalICs  ExternalResetVariant=ExternalReset  TRSumVariant=Passthrough  SumFdbkVariant=Disabled  SumVariant=Sum_PI  TsampFilterVariant=InternalTs  TsampNgainVariant=Passthrough  TsampIntegralVariant=Disabled_SignalSpec  ExternalSaturationOutDataTypeStr=Inherit: Same as second input  DerivativeSourceVariant=Disabled  PreIntVariant=InternalPreInt
  Saturation{,1..3} (4 alike) : Saturate  UpperLimit=272  LowerLimit=-272
  Scope : Scope  NumInputPorts=2
      settings: ActiveDisplayYMinimum=-0.50304569723956016  ActiveDisplayYMaximum=0.21999259282743192  DataLoggingVariableName=ScopeData41
  Scope1 : Scope
      settings: ActiveDisplayYMinimum=-1.1344677008853847  ActiveDisplayYMaximum=1.2470479181725942  DataLoggingVariableName=ScopeData28
  Scope2 : Scope
      settings: ActiveDisplayYMinimum=-0.50304569723956016  ActiveDisplayYMaximum=0.21999259282743192  DataLoggingVariableName=ScopeData29
  Subtract3 : Sum  Inputs=+-
  Terminator1 : Terminator
  Unary Minus : UnaryMinus
  Unary Minus1 : UnaryMinus
  y : Outport
  +Tx : Outport  Port=2
  -Tx : Outport  Port=3
  +Ty : Outport  Port=4
  -Ty : Outport  Port=5
  wires:
  w_demand_sat/1 -> Subtract3/1, Scope/1, Scope2/1
  Gain5/1 -> Unary Minus1/1, Saturation2/1  "deltaTy"
  Unary Minus/1 -> Saturation1/1
  Subtract3/1 -> PID Controller/1  "error"
  Demux1/3 -> Terminator1/1  "Mz"
  Demux1/2 -> Gain5/1  "My"
  Demux1/1 -> Gain4/1  "Mx"
  PID Controller/1 -> y/1, Demux1/1
  Gain4/1 -> Unary Minus/1, Saturation/1  "deltaTx"
  gyro/1 -> Subtract3/2, Scope1/1, Scope/2  "w_meas"
  Unary Minus1/1 -> Saturation3/1
  Saturation/1 -> +Ty/1
  Saturation1/1 -> -Ty/1
  Saturation3/1 -> +Tx/1
  Saturation2/1 -> -Tx/1
  DropDetected/1 -> PID Controller/2

== system platformController/PlatformController/PlatformController1/Altitude Controller Hover/Subsystem1/Enabled Subsystem ==
  Height : Inport
  Enable : EnablePort
  Out1 : Outport
  wires:
  Height/1 -> Out1/1

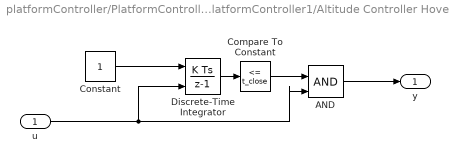
== system platformController/PlatformController/PlatformController1/Altitude Controller Hover/Subsystem1/Subsystem ==
  u : Inport
  AND : Logic  IconShape=distinctive  AllPortsSameDT=off  OutDataTypeStr=boolean
  Compare To Constant : simulink/Logic and Bit Operations/Compare To Constant  relop=<=  const=t_close  OutDataTypeStr=boolean
  Constant : Constant
  Discrete-Time Integrator : DiscreteIntegrator  ExternalReset=either  SampleTime=-1  ICPrevOutput=DiscIntNeverNeededParam  ICPrevScaledInput=DiscIntNeverNeededParam
  y : Outport
  wires:
  AND/1 -> y/1
  Constant/1 -> Discrete-Time Integrator/1
  u/1 -> Discrete-Time Integrator/2, AND/2
  Compare To Constant/1 -> AND/1
  Discrete-Time Integrator/1 -> Compare To Constant/1
